simulink model "B1_Model"  (Simulink 7.7)
settings: Solver=ode45  StartTime=0.0  StopTime=1200  MaxStep=1  RelTol=1e-3
libraries: simulink x3
settings Model: Creator=jnaber  LastModifiedBy=Arjun
settings OptimizationCC: InitFltsAndDblsToZero=on
settings DebuggingCC: SaveWithParameterizedLinksMsg=none  StrictBusMsg=Warning
settings GRTTargetCC: TargetFcnLib=ansi_tfl_tmw.mat

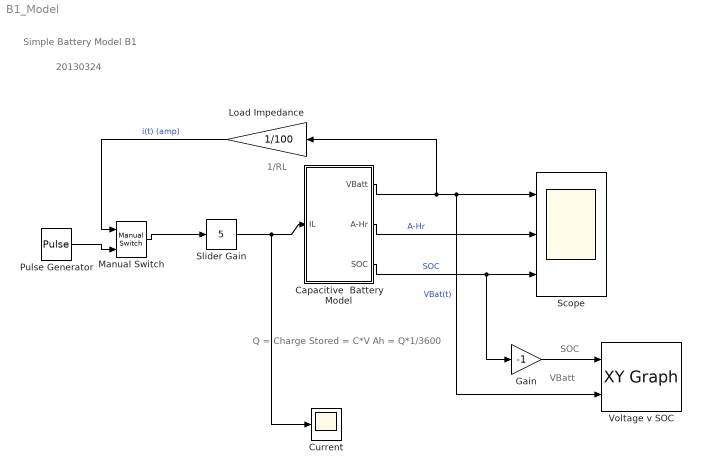
== system B1_Model ==
  note: Simple Battery Model
      | B1
  note: 20130324
  note: Q = Charge Stored  = C*V
      | Ah = Q*1/3600
  note: 1/RL
  note: SOC
  note: VBatt
  Capacitive  Battery Model : Subsystem  mask{OCV=300, RBatt=2.5, Cocv=10}
      mask prompts: OCV "Open Circuit Voltage (V)"; RBatt "Battery Resistance (Ohm)"; Cocv "Series Capacitance (F)"
  Current : Scope
  Gain : Gain  Gain=-1
  Load Impedance : Gain  Gain=1/100
  Manual Switch : simulink/Signal Routing/Manual Switch  SystemSampleTime=-1  sw=0  action=0  varsize=off
  Pulse Generator : DiscretePulseGenerator  PulseType=Time based  Period=10  PulseWidth=50  PhaseDelay=5
  Scope : Scope  NumInputPorts=3
      settings: TimeRange=4000  YMin=295.2~0~0  YMax=297~1~1  MaxDataPoints=25000  Decimation=2
  Slider Gain : simulink/Math Operations/Slider Gain  SystemSampleTime=-1  low=0  gain=5  high=50
  Voltage v SOC : simulink/Sinks/XY Graph  SystemSampleTime=-1  xmin=-1  xmax=0  ymin=0  ymax=400  st=-1
  wires:
  Capacitive  Battery Model/1(VBatt) -> Load Impedance/1, Scope/1, Voltage v SOC/2  "VBat(t)"
  Capacitive  Battery Model/3(SOC) -> Scope/3, Gain/1  "SOC"
  Capacitive  Battery Model/2(A-Hr) -> Scope/2  "A-Hr"
  Gain/1 -> Voltage v SOC/1
  Manual Switch/1 -> Slider Gain/1
  Load Impedance/1 -> Manual Switch/1  "i(t) (amp)"
  Pulse Generator/1 -> Manual Switch/2
  Slider Gain/1 -> Capacitive  Battery Model/1(IL), Current/1

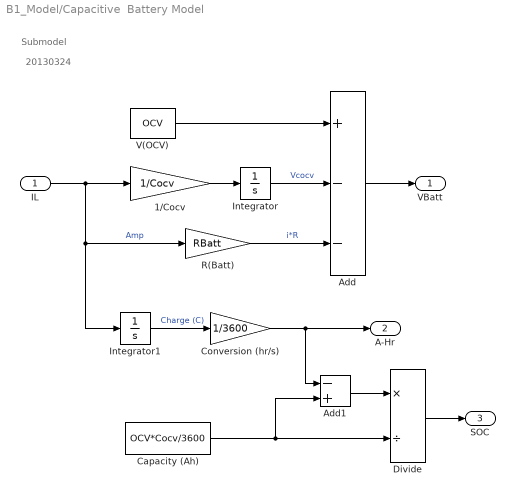
== system B1_Model/Capacitive  Battery Model ==
  note: Submodel
  note: 20130324
  IL : Inport
  1/Cocv : Gain  Gain=1/Cocv
  Add : Sum  Inputs=+--
  Add1 : Sum  Inputs=-+
  Capacity (Ah) : Constant  Value=OCV*Cocv/3600
  Conversion (hr/s) : Gain  Gain=1/3600
  Divide : Product  Inputs=*/
  Integrator : Integrator
  Integrator1 : Integrator
  R(Batt) : Gain  Gain=RBatt
  V(OCV) : Constant  Value=OCV
  VBatt : Outport
  A-Hr : Outport  Port=2
  SOC : Outport  Port=3
  wires:
  1/Cocv/1 -> Integrator/1
  V(OCV)/1 -> Add/1
  Integrator/1 -> Add/2  "Vcocv"
  R(Batt)/1 -> Add/3  "i*R"
  Add/1 -> VBatt/1
  Integrator1/1 -> Conversion (hr/s)/1  "Charge (C)"
  IL/1 -> 1/Cocv/1, R(Batt)/1, Integrator1/1  "Amp"
  Conversion (hr/s)/1 -> A-Hr/1, Add1/1
  Capacity (Ah)/1 -> Add1/2, Divide/2
  Add1/1 -> Divide/1
  Divide/1 -> SOC/1
